simulink model "benchlink"  (R2024b)
settings: Solver=FixedStepDiscrete  StartTime=0.0  StopTime=0.005*16  RelTol=1e-3
model workspace (MAT data in the model file):
  socvcb : containers.Map (value not decoded)
values from neighbouring files (symbols this model uses):
  access = [32 0 4 36 32 0 4 36 32 0 4 36 ... (16 elements, 16x1)]    [all_variables.mat]
  qam_params =     [all_variables.mat]
undefined symbols (not defined in the file or in its folder): Add, j, QAM, rms, Shift
libraries: hdlsllib x53, simulink_need_slupdate x22, simulink x18, dspsigops x16, commdigbbndam3 x6, dsphdlmathfun2 x2, commchan3 x1, commrflib2 x1, dsphdlsigops2 x1, dspstat3 x1, dsphdlfiltering2 x1, simulink_extras x1
(part 2 of 5)

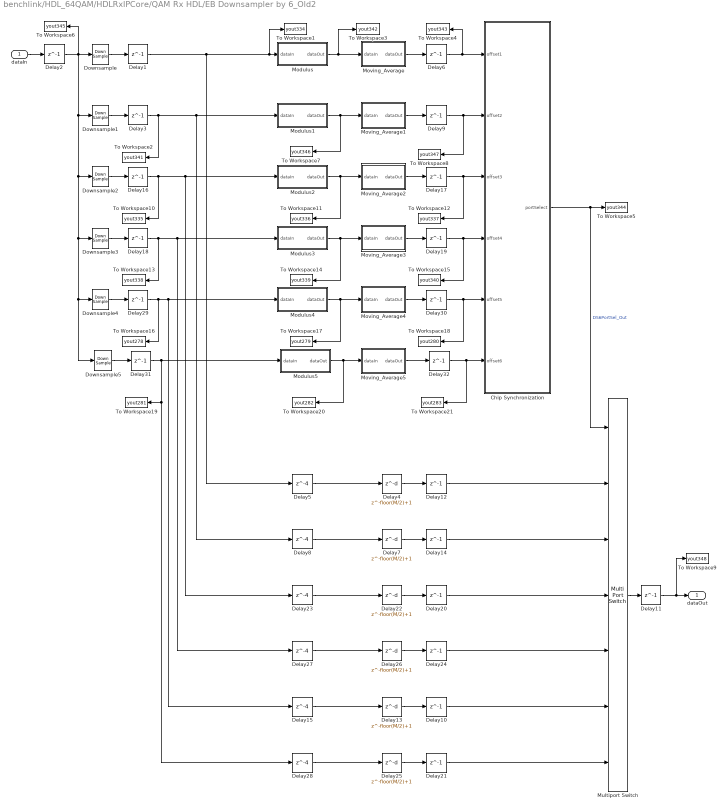
== system benchlink/HDL_64QAM/HDLRxIPCore/QAM Rx HDL/EB Downsampler by 6_Old2 ==
  dataIn : Inport  PortDimensions=1
  Chip Synchronization : MATLAB Function  TreatAsAtomicUnit=on
  Delay{1..3,6,9..12,14,16..21,24,29..32} (20 alike) : Delay  DelayLength=1  InitialCondition=0
  Delay{4,7,13,22,25..26} (6 alike) : Delay  DelayLength=floor(M/2)+1  InitialCondition=0
  Delay{5,8,15,23,27..28} (6 alike) : Delay  DelayLength=4  InitialCondition=0
  Downsample : DownSample  N=6  RateOptions=Allow multirate processing
  Downsample1 : DownSample  N=6  phase=1  RateOptions=Allow multirate processing
  Downsample2 : DownSample  N=6  phase=2  RateOptions=Allow multirate processing
  Downsample3 : DownSample  N=6  phase=3  RateOptions=Allow multirate processing
  Downsample4 : DownSample  N=6  phase=4  RateOptions=Allow multirate processing
  Downsample5 : DownSample  N=6  phase=5  RateOptions=Allow multirate processing
  Modulus : Subsystem
  Modulus1 : Subsystem
  Modulus2 : Subsystem
  Modulus3 : Subsystem
  Modulus4 : Subsystem
  Modulus5 : Subsystem
  Moving_Average : Subsystem
  Moving_Average1 : Subsystem
  Moving_Average2 : Subsystem
  Moving_Average3 : Subsystem
  Moving_Average4 : Subsystem
  Moving_Average5 : Subsystem
  Multiport Switch : MultiPortSwitch  Inputs=6  InputSameDT=off
  To Workspace1 : ToWorkspace  VariableName=yout334  SampleTime=-1
      settings: Save2DSignal=2-D array (concatenate along first dimension)
  To Workspace10 : ToWorkspace  VariableName=yout335  SampleTime=-1
      settings: Save2DSignal=2-D array (concatenate along first dimension)
  To Workspace11 : ToWorkspace  VariableName=yout336  SampleTime=-1
      settings: Save2DSignal=2-D array (concatenate along first dimension)
  To Workspace12 : ToWorkspace  VariableName=yout337  SampleTime=-1
      settings: Save2DSignal=2-D array (concatenate along first dimension)
  To Workspace13 : ToWorkspace  VariableName=yout338  SampleTime=-1
      settings: Save2DSignal=2-D array (concatenate along first dimension)
  To Workspace14 : ToWorkspace  VariableName=yout339  SampleTime=-1
      settings: Save2DSignal=2-D array (concatenate along first dimension)
  To Workspace15 : ToWorkspace  VariableName=yout340  SampleTime=-1
      settings: Save2DSignal=2-D array (concatenate along first dimension)
  To Workspace16 : ToWorkspace  VariableName=yout278  SampleTime=-1
      settings: Save2DSignal=2-D array (concatenate along first dimension)
  To Workspace17 : ToWorkspace  VariableName=yout279  SampleTime=-1
      settings: Save2DSignal=2-D array (concatenate along first dimension)
  To Workspace18 : ToWorkspace  VariableName=yout280  SampleTime=-1
      settings: Save2DSignal=2-D array (concatenate along first dimension)
  To Workspace19 : ToWorkspace  VariableName=yout281  SampleTime=-1
      settings: Save2DSignal=2-D array (concatenate along first dimension)
  To Workspace2 : ToWorkspace  VariableName=yout341  SampleTime=-1
      settings: Save2DSignal=2-D array (concatenate along first dimension)
  To Workspace20 : ToWorkspace  VariableName=yout282  SampleTime=-1
      settings: Save2DSignal=2-D array (concatenate along first dimension)
  To Workspace21 : ToWorkspace  VariableName=yout283  SampleTime=-1
      settings: Save2DSignal=2-D array (concatenate along first dimension)
  To Workspace3 : ToWorkspace  VariableName=yout342  SampleTime=-1
      settings: Save2DSignal=2-D array (concatenate along first dimension)
  To Workspace4 : ToWorkspace  VariableName=yout343  SampleTime=-1
      settings: Save2DSignal=2-D array (concatenate along first dimension)
  To Workspace5 : ToWorkspace  VariableName=yout344  SampleTime=-1
      settings: Save2DSignal=2-D array (concatenate along first dimension)
  To Workspace6 : ToWorkspace  VariableName=yout345  SampleTime=-1
      settings: Save2DSignal=2-D array (concatenate along first dimension)
  To Workspace7 : ToWorkspace  VariableName=yout346  SampleTime=-1
      settings: Save2DSignal=2-D array (concatenate along first dimension)
  To Workspace8 : ToWorkspace  VariableName=yout347  SampleTime=-1
      settings: Save2DSignal=2-D array (concatenate along first dimension)
  To Workspace9 : ToWorkspace  VariableName=yout348  SampleTime=-1
      settings: Save2DSignal=2-D array (concatenate along first dimension)
  dataOut : Outport  VectorParamsAs1DForOutWhenUnconnected=off
  wires:
  dataIn/1 -> Delay2/1
  Downsample/1 -> Delay1/1
  Modulus/1(dataOut) -> Moving_Average/1(dataIn), To Workspace3/1
  Modulus1/1(dataOut) -> Moving_Average1/1(dataIn), To Workspace7/1
  Moving_Average1/1(dataOut) -> Delay9/1
  Moving_Average/1(dataOut) -> Delay6/1
  Delay4/1 -> Delay12/1
  Delay5/1 -> Delay4/1
  Multiport Switch/1 -> Delay11/1
  Delay8/1 -> Delay7/1
  Downsample1/1 -> Delay3/1
  Delay7/1 -> Delay14/1
  Delay1/1 -> Delay5/1, To Workspace1/1, Modulus/1(dataIn)
  Delay3/1 -> To Workspace2/1, Delay8/1, Modulus1/1(dataIn)
  Delay6/1 -> To Workspace4/1, Chip Synchronization/1(offset1)
  Delay9/1 -> To Workspace8/1, Chip Synchronization/2(offset2)
  Chip Synchronization/1(portSelect) -> To Workspace5/1, Multiport Switch/1  "DS6PortSel_Out"
  Delay11/1 -> To Workspace9/1, dataOut/1
  Delay16/1 -> To Workspace10/1, Delay23/1, Modulus2/1(dataIn)
  Modulus2/1(dataOut) -> Moving_Average2/1(dataIn), To Workspace11/1
  Moving_Average2/1(dataOut) -> Delay17/1
  Delay17/1 -> To Workspace12/1, Chip Synchronization/3(offset3)
  Downsample2/1 -> Delay16/1
  Delay18/1 -> To Workspace13/1, Delay27/1, Modulus3/1(dataIn)
  Modulus3/1(dataOut) -> Moving_Average3/1(dataIn), To Workspace14/1
  Delay19/1 -> To Workspace15/1, Chip Synchronization/4(offset4)
  Downsample3/1 -> Delay18/1
  Moving_Average3/1(dataOut) -> Delay19/1
  Delay2/1 -> Downsample5/1, Downsample4/1, Downsample3/1, Downsample2/1, Downsample1/1, To Workspace6/1, Downsample/1
  Delay22/1 -> Delay20/1
  Delay23/1 -> Delay22/1
  Delay26/1 -> Delay24/1
  Delay27/1 -> Delay26/1
  Delay24/1 -> Multiport Switch/5
  Delay20/1 -> Multiport Switch/4
  Delay14/1 -> Multiport Switch/3
  Delay12/1 -> Multiport Switch/2
  Delay15/1 -> Delay13/1
  Delay13/1 -> Delay10/1
  Delay10/1 -> Multiport Switch/6
  Delay28/1 -> Delay25/1
  Delay25/1 -> Delay21/1
  Delay21/1 -> Multiport Switch/7
  Delay29/1 -> To Workspace16/1, Delay15/1, Modulus4/1(dataIn)
  Downsample4/1 -> Delay29/1
  Modulus4/1(dataOut) -> Moving_Average4/1(dataIn), To Workspace17/1
  Delay30/1 -> To Workspace18/1, Chip Synchronization/5(offset5)
  Moving_Average4/1(dataOut) -> Delay30/1
  Delay31/1 -> To Workspace19/1, Delay28/1, Modulus5/1(dataIn)
  Downsample5/1 -> Delay31/1
  Modulus5/1(dataOut) -> Moving_Average5/1(dataIn), To Workspace20/1
  Delay32/1 -> To Workspace21/1, Chip Synchronization/6(offset6)
  Moving_Average5/1(dataOut) -> Delay32/1

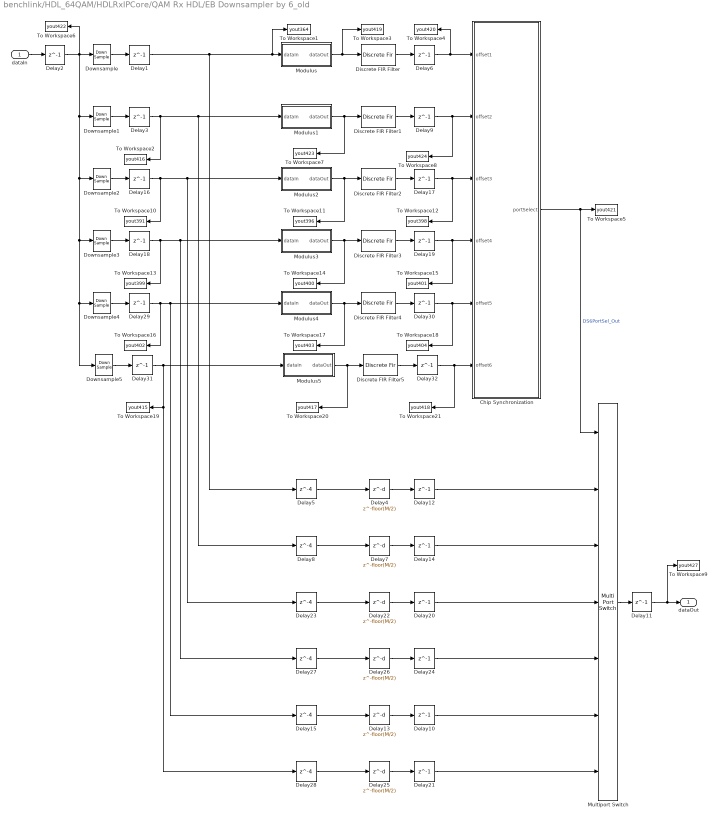
== system benchlink/HDL_64QAM/HDLRxIPCore/QAM Rx HDL/EB Downsampler by 6_old ==
  dataIn : Inport  PortDimensions=1
  Chip Synchronization : MATLAB Function  TreatAsAtomicUnit=on
  Delay{1..3,6,9..12,14,16..21,24,29..32} (20 alike) : Delay  DelayLength=1  InitialCondition=0
  Delay{4,7,13,22,25..26} (6 alike) : Delay  DelayLength=floor(M/2)  InitialCondition=0
  Delay{5,8,15,23,27..28} (6 alike) : Delay  DelayLength=4  InitialCondition=0
  Discrete FIR Filter{,1..5} (6 alike) : DiscreteFir  FilterStructure=Direct form transposed  Coefficients=ones(1,M)  CoefDataTypeStr=fixdt(1,2,0)  ProductDataTypeStr=fixdt(1,16,14)  AccumDataTypeStr=fixdt(1,16,16-floor(log2(M)+2))  OutDataTypeStr=fixdt(1,16,16-floor(log2(M)+2))  SaturateOnIntegerOverflow=on
  Downsample : DownSample  N=6  RateOptions=Allow multirate processing
  Downsample1 : DownSample  N=6  phase=1  RateOptions=Allow multirate processing
  Downsample2 : DownSample  N=6  phase=2  RateOptions=Allow multirate processing
  Downsample3 : DownSample  N=6  phase=3  RateOptions=Allow multirate processing
  Downsample4 : DownSample  N=6  phase=4  RateOptions=Allow multirate processing
  Downsample5 : DownSample  N=6  phase=5  RateOptions=Allow multirate processing
  Modulus : Subsystem
  Modulus1 : Subsystem
  Modulus2 : Subsystem
  Modulus3 : Subsystem
  Modulus4 : Subsystem
  Modulus5 : Subsystem
  Multiport Switch : MultiPortSwitch  Inputs=6  InputSameDT=off
  To Workspace1 : ToWorkspace  VariableName=yout364  SampleTime=-1
      settings: Save2DSignal=2-D array (concatenate along first dimension)
  To Workspace10 : ToWorkspace  VariableName=yout391  SampleTime=-1
      settings: Save2DSignal=2-D array (concatenate along first dimension)
  To Workspace11 : ToWorkspace  VariableName=yout396  SampleTime=-1
      settings: Save2DSignal=2-D array (concatenate along first dimension)
  To Workspace12 : ToWorkspace  VariableName=yout398  SampleTime=-1
      settings: Save2DSignal=2-D array (concatenate along first dimension)
  To Workspace13 : ToWorkspace  VariableName=yout399  SampleTime=-1
      settings: Save2DSignal=2-D array (concatenate along first dimension)
  To Workspace14 : ToWorkspace  VariableName=yout400  SampleTime=-1
      settings: Save2DSignal=2-D array (concatenate along first dimension)
  To Workspace15 : ToWorkspace  VariableName=yout401  SampleTime=-1
      settings: Save2DSignal=2-D array (concatenate along first dimension)
  To Workspace16 : ToWorkspace  VariableName=yout402  SampleTime=-1
      settings: Save2DSignal=2-D array (concatenate along first dimension)
  To Workspace17 : ToWorkspace  VariableName=yout403  SampleTime=-1
      settings: Save2DSignal=2-D array (concatenate along first dimension)
  To Workspace18 : ToWorkspace  VariableName=yout404  SampleTime=-1
      settings: Save2DSignal=2-D array (concatenate along first dimension)
  To Workspace19 : ToWorkspace  VariableName=yout415  SampleTime=-1
      settings: Save2DSignal=2-D array (concatenate along first dimension)
  To Workspace2 : ToWorkspace  VariableName=yout416  SampleTime=-1
      settings: Save2DSignal=2-D array (concatenate along first dimension)
  To Workspace20 : ToWorkspace  VariableName=yout417  SampleTime=-1
      settings: Save2DSignal=2-D array (concatenate along first dimension)
  To Workspace21 : ToWorkspace  VariableName=yout418  SampleTime=-1
      settings: Save2DSignal=2-D array (concatenate along first dimension)
  To Workspace3 : ToWorkspace  VariableName=yout419  SampleTime=-1
      settings: Save2DSignal=2-D array (concatenate along first dimension)
  To Workspace4 : ToWorkspace  VariableName=yout420  SampleTime=-1
      settings: Save2DSignal=2-D array (concatenate along first dimension)
  To Workspace5 : ToWorkspace  VariableName=yout421  SampleTime=-1
      settings: Save2DSignal=2-D array (concatenate along first dimension)
  To Workspace6 : ToWorkspace  VariableName=yout422  SampleTime=-1
      settings: Save2DSignal=2-D array (concatenate along first dimension)
  To Workspace7 : ToWorkspace  VariableName=yout423  SampleTime=-1
      settings: Save2DSignal=2-D array (concatenate along first dimension)
  To Workspace8 : ToWorkspace  VariableName=yout424  SampleTime=-1
      settings: Save2DSignal=2-D array (concatenate along first dimension)
  To Workspace9 : ToWorkspace  VariableName=yout427  SampleTime=-1
      settings: Save2DSignal=2-D array (concatenate along first dimension)
  dataOut : Outport  VectorParamsAs1DForOutWhenUnconnected=off
  wires:
  dataIn/1 -> Delay2/1
  Downsample/1 -> Delay1/1
  Modulus/1(dataOut) -> To Workspace3/1, Discrete FIR Filter/1
  Modulus1/1(dataOut) -> To Workspace7/1, Discrete FIR Filter1/1
  Discrete FIR Filter1/1 -> Delay9/1
  Discrete FIR Filter/1 -> Delay6/1
  Delay4/1 -> Delay12/1
  Delay5/1 -> Delay4/1
  Multiport Switch/1 -> Delay11/1
  Delay8/1 -> Delay7/1
  Downsample1/1 -> Delay3/1
  Delay7/1 -> Delay14/1
  Delay1/1 -> Delay5/1, To Workspace1/1, Modulus/1(dataIn)
  Delay3/1 -> To Workspace2/1, Delay8/1, Modulus1/1(dataIn)
  Delay6/1 -> To Workspace4/1, Chip Synchronization/1(offset1)
  Delay9/1 -> To Workspace8/1, Chip Synchronization/2(offset2)
  Chip Synchronization/1(portSelect) -> To Workspace5/1, Multiport Switch/1  "DS6PortSel_Out"
  Delay11/1 -> To Workspace9/1, dataOut/1
  Delay16/1 -> To Workspace10/1, Delay23/1, Modulus2/1(dataIn)
  Modulus2/1(dataOut) -> To Workspace11/1, Discrete FIR Filter2/1
  Discrete FIR Filter2/1 -> Delay17/1
  Delay17/1 -> To Workspace12/1, Chip Synchronization/3(offset3)
  Downsample2/1 -> Delay16/1
  Delay18/1 -> To Workspace13/1, Delay27/1, Modulus3/1(dataIn)
  Modulus3/1(dataOut) -> To Workspace14/1, Discrete FIR Filter3/1
  Delay19/1 -> To Workspace15/1, Chip Synchronization/4(offset4)
  Downsample3/1 -> Delay18/1
  Discrete FIR Filter3/1 -> Delay19/1
  Delay2/1 -> Downsample5/1, Downsample4/1, Downsample3/1, Downsample2/1, Downsample1/1, To Workspace6/1, Downsample/1
  Delay22/1 -> Delay20/1
  Delay23/1 -> Delay22/1
  Delay26/1 -> Delay24/1
  Delay27/1 -> Delay26/1
  Delay24/1 -> Multiport Switch/5
  Delay20/1 -> Multiport Switch/4
  Delay14/1 -> Multiport Switch/3
  Delay12/1 -> Multiport Switch/2
  Delay15/1 -> Delay13/1
  Delay13/1 -> Delay10/1
  Delay10/1 -> Multiport Switch/6
  Delay28/1 -> Delay25/1
  Delay25/1 -> Delay21/1
  Delay21/1 -> Multiport Switch/7
  Delay29/1 -> To Workspace16/1, Delay15/1, Modulus4/1(dataIn)
  Downsample4/1 -> Delay29/1
  Modulus4/1(dataOut) -> To Workspace17/1, Discrete FIR Filter4/1
  Delay30/1 -> To Workspace18/1, Chip Synchronization/5(offset5)
  Discrete FIR Filter4/1 -> Delay30/1
  Delay31/1 -> To Workspace19/1, Delay28/1, Modulus5/1(dataIn)
  Downsample5/1 -> Delay31/1
  Modulus5/1(dataOut) -> To Workspace20/1, Discrete FIR Filter5/1
  Delay32/1 -> To Workspace21/1, Chip Synchronization/6(offset6)
  Discrete FIR Filter5/1 -> Delay32/1

== system benchlink/HDL_64QAM/HDLRxIPCore/QAM Rx HDL/EQ Enable ==
  EQEnable : Inport
  Constant19 : Constant  OutDataTypeStr=boolean  SampleTime=1/(qam_params.chipRate)
  Constant20 : Constant  Value=0  OutDataTypeStr=boolean  SampleTime=1/(qam_params.chipRate)
  Switch9 : Switch  Criteria=u2 ~= 0  SaturateOnIntegerOverflow=off  InputSameDT=off
  Unit Delay : UnitDelay  InitialCondition=int16(150)  SampleTime=-1  HasFrameUpgradeWarning=on
  Out : Outport  VectorParamsAs1DForOutWhenUnconnected=off
  wires:
  EQEnable/1 -> Unit Delay/1
  Constant19/1 -> Switch9/1
  Unit Delay/1 -> Switch9/2
  Constant20/1 -> Switch9/3
  Switch9/1 -> Out/1

== system benchlink/HDL_64QAM/HDLRxIPCore/QAM Rx HDL/Enabled AGC1 ==
  x : Inport
  AGCEnable : Inport  Port=2  PortDimensions=1
  Constant : Constant  OutDataTypeStr=fixdt(1,24,15)  SampleTime=1/(qam_params.sampleRate)
  Delay : Delay  InitialCondition=0
  Delay1 : Delay  InitialCondition=0
  Delay2 : Delay  DelayLength=1  InitialCondition=0
  Delay3 : Delay  DelayLength=1  InitialCondition=0
  Delay4 : Delay  InitialCondition=0
  Energy Detector : Subsystem
  Loop gain : Constant  Value=AGC_Gain  OutDataTypeStr=fixdt(1,16,15)  SampleTime=1/qam_params.sampleRate
  Product : Product  OutDataTypeStr=fixdt(1,16,15)  SaturateOnIntegerOverflow=on
  Product1 : Product  OutDataTypeStr=fixdt(1,16,15)  SaturateOnIntegerOverflow=on
  Reference : Constant  Value=AGC_Ref  OutDataTypeStr=fixdt(1,16,15)  SampleTime=1/qam_params.sampleRate
  Sum : Sum  OutDataTypeStr=Inherit: Same as accumulator  AccumDataTypeStr=fixdt(1,24,15)  SaturateOnIntegerOverflow=on
  Sum1 : Sum  Inputs=|-+  OutDataTypeStr=Inherit: Same as first input
  Switch9 : Switch  Criteria=u2 ~= 0  SaturateOnIntegerOverflow=off  InputSameDT=off
  To Workspace1 : ToWorkspace  VariableName=yout471  SampleTime=-1
      settings: Save2DSignal=2-D array (concatenate along first dimension)
  To Workspace8 : ToWorkspace  VariableName=yout472  SampleTime=-1
      settings: Save2DSignal=2-D array (concatenate along first dimension)
  Unit Delay : UnitDelay  InitialCondition=.5  SampleTime=-1  HasFrameUpgradeWarning=on
  Unit Delay Enabled : simulink_need_slupdate/Unit Delay Enabled  vinit=1  tsamp=-1
  power : Subsystem
  gain : Outport  VectorParamsAs1DForOutWhenUnconnected=off
  y : Outport  Port=2  PortDimensions=1  VectorParamsAs1DForOutWhenUnconnected=off
  wires:
  Product/1 -> Delay/1
  Sum1/1 -> Delay2/1  "e"
  Delay2/1 -> Product1/1
  Product1/1 -> Delay4/1
  Unit Delay/1 -> gain/1, Switch9/1, Unit Delay Enabled/1  "g"
  Delay4/1 -> Sum/2
  x/1 -> Delay1/1
  Loop gain/1 -> Product1/2
  Sum/1 -> Unit Delay/1
  Reference/1 -> Sum1/2
  Delay1/1 -> To Workspace8/1, Product/1, Energy Detector/1(In)
  Delay/1 -> power/1(In1), y/1
  power/1(Out1) -> Sum1/1  "magnew"
  Energy Detector/1(Out) -> To Workspace1/1, Unit Delay Enabled/2
  Unit Delay Enabled/1 -> Sum/1
  Delay3/1 -> Switch9/2
  AGCEnable/1 -> Delay3/1
  Constant/1 -> Switch9/3
  Switch9/1 -> Product/2

== system benchlink/HDL_64QAM/HDLRxIPCore/QAM Rx HDL/Enabled AGC2 ==
  x : Inport
  AGCEnable : Inport  Port=2  PortDimensions=1
  Constant : Constant  OutDataTypeStr=fixdt(1,24,15)  SampleTime=1/(qam_params.sampleRate)
  Delay : Delay  InitialCondition=0
  Delay1 : Delay  InitialCondition=0
  Delay2 : Delay  DelayLength=1  InitialCondition=0
  Delay3 : Delay  DelayLength=1  InitialCondition=0
  Delay4 : Delay  InitialCondition=0
  Energy Detector : Subsystem
  Loop gain : Constant  Value=AGC_Gain  OutDataTypeStr=fixdt(1,16,15)  SampleTime=1/qam_params.sampleRate
  Product : Product  OutDataTypeStr=fixdt(1,16,15)  SaturateOnIntegerOverflow=on
  Product1 : Product  OutDataTypeStr=fixdt(1,16,15)  SaturateOnIntegerOverflow=on
  Reference : Constant  Value=AGC_Ref  OutDataTypeStr=fixdt(1,16,15)  SampleTime=1/qam_params.sampleRate
  Sum : Sum  OutDataTypeStr=Inherit: Same as accumulator  AccumDataTypeStr=fixdt(1,24,15)  SaturateOnIntegerOverflow=on
  Sum1 : Sum  Inputs=|-+  OutDataTypeStr=Inherit: Same as first input
  Switch9 : Switch  Criteria=u2 ~= 0  SaturateOnIntegerOverflow=off  InputSameDT=off
  Unit Delay : UnitDelay  InitialCondition=.5  SampleTime=-1  HasFrameUpgradeWarning=on
  Unit Delay Enabled : simulink_need_slupdate/Unit Delay Enabled  vinit=1  tsamp=-1
  power : Subsystem
  signal power1 : Subsystem
  gain : Outport  VectorParamsAs1DForOutWhenUnconnected=off
  y : Outport  Port=2  PortDimensions=1  VectorParamsAs1DForOutWhenUnconnected=off
  sig_power : Outport  Port=3  PortDimensions=1  VectorParamsAs1DForOutWhenUnconnected=off
  wires:
  Product/1 -> Delay/1
  Sum1/1 -> Delay2/1  "e"
  Delay2/1 -> Product1/1
  Product1/1 -> Delay4/1
  Delay4/1 -> Sum/2
  x/1 -> Delay1/1
  Loop gain/1 -> Product1/2
  Sum/1 -> Unit Delay/1
  Reference/1 -> Sum1/2
  Delay1/1 -> signal power1/1(x), Product/1, Energy Detector/1(In)
  Delay/1 -> power/1(In1), y/1
  power/1(Out1) -> Sum1/1  "magnew"
  Energy Detector/1(trigger) -> signal power1/2(trigger), Unit Delay Enabled/2
  Unit Delay Enabled/1 -> Sum/1
  AGCEnable/1 -> Delay3/1
  Delay3/1 -> Switch9/2
  Constant/1 -> Switch9/3
  Unit Delay/1 -> Unit Delay Enabled/1, Switch9/1, gain/1  "g"
  Switch9/1 -> Product/2
  signal power1/1(signal_power) -> sig_power/1

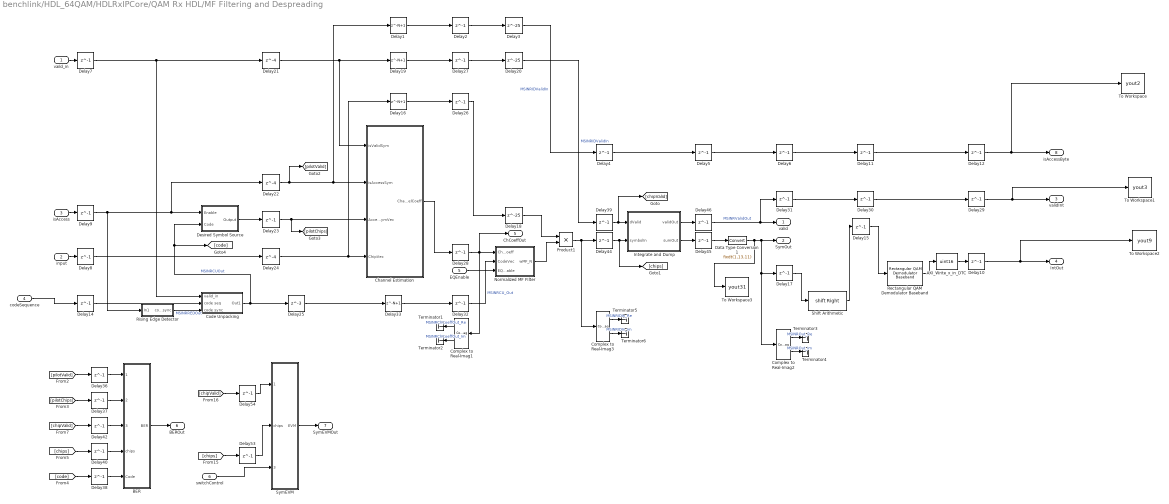
== system benchlink/HDL_64QAM/HDLRxIPCore/QAM Rx HDL/MF Filtering and Despreading ==
  vaild_in : Inport
  input : Inport  Port=2
  isAccess : Inport  Port=3
  codeSequence : Inport  Port=4
  EQEnable : Inport  Port=5
  switchControl : Inport  Port=6
  " Integrate and Dump" : MATLAB Function  TreatAsAtomicUnit=on
  AXI_Write_x_in_DTC : DataTypeConversion  OutDataTypeStr=uint16  ConvertRealWorld=Stored Integer (SI)  SaturateOnIntegerOverflow=off  RndMeth=Floor
  BER : Subsystem
  Channel Estimation : Subsystem
  Code Unpacking : Subsystem
  Complex to Real-Imag1 : ComplexToRealImag
  Complex to Real-Imag2 : ComplexToRealImag
  Complex to Real-Imag3 : ComplexToRealImag
  Data Type Conversion1 : DataTypeConversion  OutDataTypeStr=fixdt(1,13,11)  RndMeth=Floor
  Delay{1,16,19,33} (4 alike) : Delay  DelayLength=N+1  InitialCondition=0
  Delay{2,4..12,14..15,17,23,26..32,36..40,42,44..46,53..54} (32 alike) : Delay  DelayLength=1  InitialCondition=0
  Delay18 : Delay  DelayLength=25  InitialCondition=0
  Delay20 : Delay  DelayLength=25  InitialCondition=0
  Delay21 : Delay  DelayLength=4  InitialCondition=0
  Delay22 : Delay  DelayLength=4  InitialCondition=0
  Delay24 : Delay  DelayLength=4  InitialCondition=0
  Delay25 : Delay  DelayLength=3  InitialCondition=0
  Delay3 : Delay  DelayLength=25  InitialCondition=0
  Desired Symbol Source : Subsystem
  Normalized MF FIlter : Subsystem
  Product1 : Product  OutDataTypeStr=fixdt(1,16,14)  RndMeth=Zero  SaturateOnIntegerOverflow=on
  Rectangular QAM Demodulator Baseband : commdigbbndam3/Rectangular QAM Demodulator Baseband  M=64  OutType=Integer  DecType=Hard decision  VarSource=Dialog  Variance=1  Dec=Gray  Mapping=[0:15]  PowType=Min. distance between symbols  MinDist=2  AvgPow=0.66  PeakPow=1  Ph=0  outDtype1=boolean  outDtype2=Inherit via internal rule  derotateFactorWordLen=16  derotateFactorDataTypeStr=Inherit: Same word length as input  derotateFactorLastDataTypeStr=Inherit: Same word length as input  denormFactorWordLen=16  denormFactorDataTypeStr=Inherit: Same word length as input  denormFactorLastDataTypeStr=Inherit: Same word length as input  prodOutWordLen=32  prodOutOverflowMode=Wrap  prodOutRoundingMode=Floor  prodOutOvFlMode=off  prodOutOvFlModeLastStrValue=off  sumWordLen=32
  Rising Edge Detector : Subsystem
  Shift Arithmetic : ArithShift  BinPtShiftNumber=3  BitShiftDirection=Right
  SymEVM : Subsystem
  Terminator{1..6} (6 alike) : Terminator
  To Workspace : ToWorkspace  VariableName=yout2  SampleTime=-1
      settings: Save2DSignal=2-D array (concatenate along first dimension)
  To Workspace1 : ToWorkspace  VariableName=yout3  SampleTime=-1
      settings: Save2DSignal=2-D array (concatenate along first dimension)
  To Workspace2 : ToWorkspace  VariableName=yout9  SampleTime=-1
      settings: Save2DSignal=2-D array (concatenate along first dimension)
  To Workspace3 : ToWorkspace  VariableName=yout31  SampleTime=-1
      settings: Save2DSignal=2-D array (concatenate along first dimension)
  valid : Outport  InitialOutput=0  VectorParamsAs1DForOutWhenUnconnected=off
  SymOut : Outport  Port=2  InitialOutput=0  VectorParamsAs1DForOutWhenUnconnected=off
  validInt : Outport  Port=3  InitialOutput=0  VectorParamsAs1DForOutWhenUnconnected=off
  IntOut : Outport  Port=4  InitialOutput=0  VectorParamsAs1DForOutWhenUnconnected=off
  ChCoeffOut : Outport  Port=5  InitialOutput=0  VectorParamsAs1DForOutWhenUnconnected=off
  BEROut : Outport  Port=6  InitialOutput=0  VectorParamsAs1DForOutWhenUnconnected=off
  SymEVMOut : Outport  Port=7  InitialOutput=0  VectorParamsAs1DForOutWhenUnconnected=off
  isAccessByte : Outport  Port=8  InitialOutput=0  VectorParamsAs1DForOutWhenUnconnected=off
  wires:
  Delay14/1 -> Code Unpacking/2(code seq)
  vaild_in/1 -> Delay7/1
  input/1 -> Delay8/1
  codeSequence/1 -> Delay14/1
  isAccess/1 -> Delay9/1
  Desired Symbol Source/1(Output) -> Delay23/1
  Delay8/1 -> Delay24/1
  Delay9/1 -> Rising Edge Detector/1(In1), Desired Symbol Source/1(Enable), Delay22/1
  Channel Estimation/1(ChannelCoeff) -> Delay28/1
  Delay16/1 -> Delay26/1
  Code Unpacking/1(Out1) -> Delay25/1, [code], Desired Symbol Source/2(Code)  "MSINRCUOut"
  Delay19/1 -> Delay27/1
  Delay20/1 -> Delay39/1  "MSINRIDValidIn"
  Delay7/1 -> Code Unpacking/1(valid_in), Delay21/1
  Delay18/1 -> Product1/1
  Normalized MF FIlter/1(wMF_N) -> Product1/2
  Delay21/1 -> Delay19/1, Channel Estimation/1(isValidSym)
  Delay24/1 -> Delay16/1, Channel Estimation/4(ChipVec)
  Delay25/1 -> Delay33/1
  Delay26/1 -> Delay18/1
  Delay27/1 -> Delay20/1
  Delay28/1 -> ChCoeffOut/1, Complex to Real-Imag1/1, Normalized MF FIlter/1(ChannelCoeff)
  Shift Arithmetic/1 -> Delay15/1
  Delay15/1 -> Rectangular QAM Demodulator Baseband/1
  Rectangular QAM Demodulator Baseband/1 -> AXI_Write_x_in_DTC/1
  Delay17/1 -> Shift Arithmetic/1
  Delay10/1 -> To Workspace2/1, IntOut/1
  Delay29/1 -> To Workspace1/1, validInt/1
  Delay31/1 -> Delay30/1
  Delay30/1 -> Delay29/1
  Rising Edge Detector/1(code sync) -> Code Unpacking/3(code sync)  "MSINRREDOut"
  Delay45/1 -> Data Type Conversion1/1
  Product1/1 -> Complex to Real-Imag3/1, Delay44/1
  " Integrate and Dump"/1(validOut) -> Delay46/1
  " Integrate and Dump"/2(sumOut) -> Delay45/1
  Data Type Conversion1/1 -> To Workspace3/1, SymOut/1, Complex to Real-Imag2/1, Delay17/1
  Delay46/1 -> valid/1, Delay31/1  "MSINRValidOut"
  Delay32/1 -> Normalized MF FIlter/2(CodeVec)  "MSINRCU_Out"
  Complex to Real-Imag2/2 -> Terminator4/1  "MSINROut_Im"
  Complex to Real-Imag2/1 -> Terminator3/1  "MSINROut_Re"
  Complex to Real-Imag1/1 -> Terminator1/1  "MSINRChCoeffOut_Re"
  Complex to Real-Imag1/2 -> Terminator2/1  "MSINRChCoeffOut_Im"
  Complex to Real-Imag3/2 -> Terminator6/1  "MSINRIDIn_Im"
  Complex to Real-Imag3/1 -> Terminator5/1  "MSINRIDIn_Re"
  Delay33/1 -> Delay32/1
  EQEnable/1 -> Normalized MF FIlter/3(EQEnable)
  Delay54/1 -> SymEVM/1(chipValid)
  [chipValid] -> Delay54/1
  Delay53/1 -> SymEVM/2(chips)
  [pilotValid] -> Delay36/1
  [chips] -> Delay53/1
  Delay42/1 -> BER/3(chipValid)
  SymEVM/1(EVM) -> SymEVMOut/1
  [code] -> Delay38/1
  [pilotChips] -> Delay37/1
  Delay38/1 -> BER/5(Code)
  [chips] -> Delay40/1
  Delay37/1 -> BER/2(pilotChips)
  BER/1(BER) -> BEROut/1
  [chipValid] -> Delay42/1
  Delay40/1 -> BER/4(chips)
  Delay36/1 -> BER/1(pilotValid)
  Delay23/1 -> [pilotChips], Channel Estimation/3(AccessSymVec)
  Delay44/1 -> [chips], " Integrate and Dump"/2(symbolIn)
  Delay39/1 -> " Integrate and Dump"/1(dValid), [chipValid]
  Delay22/1 -> [pilotValid], Delay1/1, Channel Estimation/2(isAccessSym)
  AXI_Write_x_in_DTC/1 -> Delay10/1
  Delay1/1 -> Delay2/1
  Delay2/1 -> Delay3/1
  Delay3/1 -> Delay4/1  "MSINRIDValidIn"
  Delay4/1 -> Delay5/1
  Delay5/1 -> Delay6/1
  Delay6/1 -> Delay11/1
  Delay11/1 -> Delay12/1
  Delay12/1 -> To Workspace/1, isAccessByte/1
  switchControl/1 -> SymEVM/3(switchControl)

== system benchlink/HDL_64QAM/HDLRxIPCore/QAM Rx HDL/PD Threshold ==
  PDThreshold : Inport
  Bit Concat : hdlsllib/Logic and Bit Operations/Bit Concat  numInputs=7
  Bit Slice : hdlsllib/Logic and Bit Operations/Bit Slice  lidx=5  ridx=5
  Bit Slice1 : hdlsllib/Logic and Bit Operations/Bit Slice  lidx=4  ridx=4
  Bit Slice2 : hdlsllib/Logic and Bit Operations/Bit Slice  lidx=3  ridx=3
  Bit Slice3 : hdlsllib/Logic and Bit Operations/Bit Slice  lidx=2  ridx=2
  Bit Slice4 : hdlsllib/Logic and Bit Operations/Bit Slice  lidx=1  ridx=1
  Bit Slice5 : hdlsllib/Logic and Bit Operations/Bit Slice  lidx=0  ridx=0
  Bit Slice6 : hdlsllib/Logic and Bit Operations/Bit Slice  lidx=6  ridx=6
  Constant{6,8,10,12,14,16,18} (7 alike) : Constant  Value=0  OutDataTypeStr=boolean  SampleTime=1/(qam_params.chipRate)
  Constant{5,7,9,11,13,15,17} (7 alike) : Constant  OutDataTypeStr=boolean  SampleTime=1/(qam_params.chipRate)
  Scale : Gain  Gain=0.01  OutDataTypeStr=fixdt(0,16,15)  RndMeth=Zero
  Switch{1..7} (7 alike) : Switch  Criteria=u2 ~= 0  SaturateOnIntegerOverflow=off  InputSameDT=off
  Unit Delay : UnitDelay  InitialCondition=int16(150)  SampleTime=-1  HasFrameUpgradeWarning=on
  Out : Outport  VectorParamsAs1DForOutWhenUnconnected=off
  wires:
  Constant16/1 -> Switch6/3
  Bit Slice3/1 -> Switch5/2
  Constant17/1 -> Switch7/1
  Constant14/1 -> Switch5/3
  Bit Slice1/1 -> Switch3/2
  Constant13/1 -> Switch5/1
  Bit Slice4/1 -> Switch6/2
  Constant11/1 -> Switch4/1
  Bit Slice/1 -> Switch2/2
  Constant10/1 -> Switch3/3
  Bit Slice5/1 -> Switch7/2
  Bit Slice2/1 -> Switch4/2
  Constant18/1 -> Switch7/3
  Constant12/1 -> Switch4/3
  Constant6/1 -> Switch1/3
  Constant7/1 -> Switch2/1
  Constant15/1 -> Switch6/1
  Constant9/1 -> Switch3/1
  Bit Slice6/1 -> Switch1/2
  Constant5/1 -> Switch1/1
  Constant8/1 -> Switch2/3
  PDThreshold/1 -> Unit Delay/1
  Bit Concat/1 -> Scale/1
  Unit Delay/1 -> Bit Slice6/1, Bit Slice/1, Bit Slice1/1, Bit Slice2/1, Bit Slice3/1, Bit Slice4/1, Bit Slice5/1
  Scale/1 -> Out/1
  Switch1/1 -> Bit Concat/1
  Switch7/1 -> Bit Concat/7
  Switch6/1 -> Bit Concat/6
  Switch5/1 -> Bit Concat/5
  Switch4/1 -> Bit Concat/4
  Switch3/1 -> Bit Concat/3
  Switch2/1 -> Bit Concat/2

== system benchlink/HDL_64QAM/HDLRxIPCore/QAM Rx HDL/Payload Delimiter ==
  Input : Inport
  Threshold : Inport  Port=2
  fineCorrections : Inport  Port=3
  switchControl : Inport  Port=4
  packetSymLength : Inport  Port=5
  Constant : Constant  Commented=on  Value=threshold  OutDataTypeStr=Inherit: Inherit via back propagation  SampleTime=1/qam_params.chipRate
  Data Type Conversion1 : DataTypeConversion  RndMeth=Floor
  Delay{1..2,4..7,9..13} (11 alike) : Delay  DelayLength=1  InitialCondition=0
  For Normalized Modulus w Golay : Delay  DelayLength=7  InitialCondition=0
  MATLAB Function1 : MATLAB Function  TreatAsAtomicUnit=on
  MATLAB Function2 : MATLAB Function  Commented=on  TreatAsAtomicUnit=on
  Normalized Modulus : Subsystem
  Peak Detector : Subsystem
  Preamble Matched Filter : Subsystem
  Relational Operator : RelationalOperator  OutDataTypeStr=boolean
  Rising Edge Detector : Subsystem
  ffcControl : MATLAB Function  TreatAsAtomicUnit=on
  frameIndexing : Subsystem
  valid : Outport  InitialOutput=0  VectorParamsAs1DForOutWhenUnconnected=off
  output : Outport  Port=2  InitialOutput=0  VectorParamsAs1DForOutWhenUnconnected=off
  isAccess : Outport  Port=3  InitialOutput=0  VectorParamsAs1DForOutWhenUnconnected=off
  AccessStart : Outport  Port=4  InitialOutput=0  VectorParamsAs1DForOutWhenUnconnected=off
  wires:
  MATLAB Function1/1(isValid) -> Delay2/1
  MATLAB Function1/2(isAccess) -> Delay1/1
  Threshold/1 -> Data Type Conversion1/1
  Input/1 -> Delay12/1
  Delay2/1 -> valid/1
  Delay1/1 -> isAccess/1
  Delay11/1 -> output/1
  For Normalized Modulus w Golay/1 -> Delay5/1
  Delay9/1 -> Delay11/1
  Normalized Modulus/2(dataOutN) -> Relational Operator/1, Peak Detector/1(xCorr)  "PDNxCorrOut"
  Delay10/1 -> Delay4/1
  Delay4/1 -> AccessStart/1
  Preamble Matched Filter/1(dataOut) -> Normalized Modulus/1(dataIn)
  Relational Operator/1 -> Peak Detector/2(Threshold)
  Delay5/1 -> Delay13/1
  Data Type Conversion1/1 -> Relational Operator/2
  Peak Detector/1(Out1) -> Rising Edge Detector/1(In1), Delay6/1
  Delay6/1 -> MATLAB Function1/1(enable), Delay10/1
  Delay7/1 -> MATLAB Function1/2(count)
  Delay13/1 -> Delay9/1
  Delay12/1 -> Preamble Matched Filter/1(dataIn), For Normalized Modulus w Golay/1
  fineCorrections/1 -> ffcControl/1(correctionsPerPack)
  ffcControl/1(accessChipStart) -> MATLAB Function1/3(accessChipStart)
  Rising Edge Detector/1(Out1) -> frameIndexing/1(rst)
  frameIndexing/1(Out1) -> Delay7/1
  packetSymLength/1 -> MATLAB Function1/4(packetSymLen)
  switchControl/1 -> frameIndexing/2(switchControl), Normalized Modulus/2(switchControl)

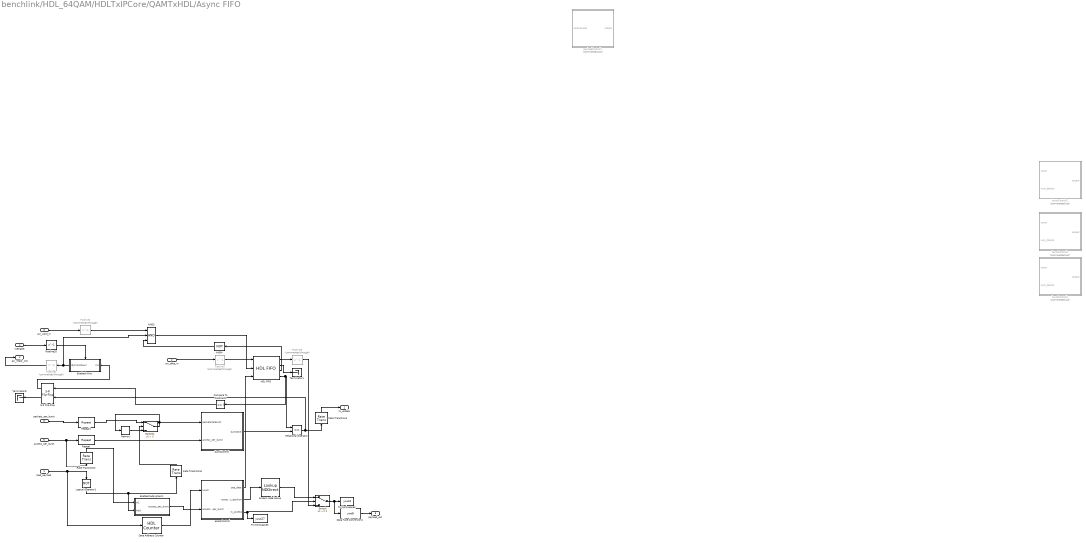
== system benchlink/HDL_64QAM/HDLTxIPCore/QAMTxHDL/Async FIFO ==
  load_payload : Inport
  axi_data_in : Inport  Port=2
  axi_valid_in : Inport  Port=3
  txEnable : Inport  Port=4
  access_per_burst : Inport  Port=5
  packets_per_burst : Inport  Port=6
  AND3 : Logic  Inputs=3  IconShape=distinctive  AllPortsSameDT=off  OutDataTypeStr=boolean
  AND4 : Logic  Operator=NOT  IconShape=distinctive  AllPortsSameDT=off  OutDataTypeStr=boolean
  Compare To Constant1 : simulink/Logic and Bit Operations/Compare To Constant  relop===  const=0  OutDataTypeStr=boolean
  Data Address Counter : hdlsllib/Sources/HDL Counter  CountType=Count limited  CountInit=0  CountStep=1  CountMax=255  CountFromType=Initial value  CountFrom=0  CountResetPort=off  CountLoadPort=off  CountEnbPort=on  CountDirPort=off  CountHitOutputPort=off  CountDataType=Unsigned  CountWordLen=16  CountFracLen=0  CountSampTime=1
  Data Type Conversion1 : DataTypeConversion  OutDataTypeStr=uint8  SaturateOnIntegerOverflow=off  RndMeth=Floor
  Enabled Subsystem1 : Subsystem  TreatAsAtomicUnit=on
  Enabled Wire : Subsystem  TreatAsAtomicUnit=on
  HDL FIFO : hdlsllib/HDL RAMs/HDL FIFO  fifo_size=2048  mode=Classic  ratio=48  push_msg=Warning  pop_msg=Warning  show_empty=on  show_full=on  show_num=on  LabelModeActiveChoice_Mode=Classic  rst_port=off
  Logical Operator1 : Logic  Operator=NOT  AllPortsSameDT=off  OutDataTypeStr=boolean
  Memory : Memory  InheritSampleTime=on
  Pipeline1 : Delay  Commented=through  DelayLength=1  InitialCondition=0  SampleTime=1/qam_params.sampleRate
  Pipeline2 : Delay  Commented=through  DelayLength=1  InitialCondition=0  SampleTime=1/qam_params.sampleRate
  Pipeline20 : Delay  DelayLength=1  InitialCondition=0
  Pipeline3 : Delay  Commented=through  DelayLength=1  InitialCondition=0  SampleTime=1/qam_params.sampleRate
  Pipeline9 : Delay  Commented=through  DelayLength=1  InitialCondition=0  SampleTime=1/qam_params.symbolRate
  Rate Transition1 : RateTransition  OutPortSampleTime=1/qam_params.symbolRate
  Rate Transition2 : RateTransition  OutPortSampleTime=1/qam_params.symbolRate
  Rate Transition3 : RateTransition  OutPortSampleTime=2.5000010000004e-08
  Relational Operator : RelationalOperator  Operator===  OutDataTypeStr=boolean  RndMeth=Simplest  InputSameDT=off
  Repeat : dspsigops/Repeat  FactorSource=Dialog parameter  N=qam_params.Upsampling  Nmax=16  InputProcessing=Columns as channels (frame based)  RateOptions=Allow multirate processing  ic=0  mode=Unused parameter value
  Repeat1 : dspsigops/Repeat  FactorSource=Dialog parameter  N=qam_params.Upsampling  Nmax=16  InputProcessing=Columns as channels (frame based)  RateOptions=Allow multirate processing  ic=0  mode=Unused parameter value
  S-R Flip-Flop : simulink_extras/Flip Flops/S-R Flip-Flop  initial_condition=0
  Switch : Switch  Criteria=u2 ~= 0  Threshold=15  SaturateOnIntegerOverflow=off  InputSameDT=off
  Switch1 : Switch  Criteria=u2 > Threshold  SaturateOnIntegerOverflow=off  InputSameDT=off
  Terminator1 : Terminator
  Terminator9 : Terminator
  To Workspace2 : ToWorkspace  VariableName=yout4  SampleTime=-1
      settings: Save2DSignal=2-D array (concatenate along first dimension)
  To Workspace3 : ToWorkspace  VariableName=yout27  SampleTime=-1
      settings: Save2DSignal=2-D array (concatenate along first dimension)
  access code lookup : LookupNDDirect  NumberOfTableDimensions=1  Table=access  DiagnosticForOutOfRangeInput=Error  TableDataTypeStr=uint32
  acessControl : MATLAB Function  TreatAsAtomicUnit=on
  burstControl : MATLAB Function  TreatAsAtomicUnit=on
  burstControl2 : MATLAB Function  Commented=on  TreatAsAtomicUnit=on
  burstControl3 : MATLAB Function  Commented=on  TreatAsAtomicUnit=on
  burstControl4 : MATLAB Function  Commented=on  TreatAsAtomicUnit=on
  payloadControl1 : MATLAB Function  Commented=on  TreatAsAtomicUnit=on  SystemSampleTime=1/qam_params.symbolRate
  tx_enable : Outport
  axi_ready_out : Outport  Port=2
  payload_out : Outport  Port=3
  wires:
  Enabled Wire/1(rdyFromDown) -> Pipeline1/1, AND3/2
  acessControl/3(is_access) -> Switch/2, To Workspace3/1
  Relational Operator/1 -> Rate Transition1/1, S-R Flip-Flop/2
  Compare To Constant1/1 -> S-R Flip-Flop/1
  Data Address Counter/1 -> acessControl/1(count)
  Pipeline3/1 -> HDL FIFO/1
  Pipeline2/1 -> AND3/1
  Pipeline1/1 -> axi_ready_out/1
  load_payload/1 -> Logical Operator1/1, Data Address Counter/1
  HDL FIFO/3 -> AND4/1
  Rate Transition1/1 -> tx_enable/1
  axi_valid_in/1 -> Pipeline2/1
  HDL FIFO/4 -> Compare To Constant1/1, Relational Operator/1
  S-R Flip-Flop/1 -> Enabled Wire/1(In1)
  axi_data_in/1 -> Pipeline3/1
  Switch/1 -> Data Type Conversion1/1, To Workspace2/1
  Rate Transition2/1 -> Enabled Subsystem1/1(In1)
  burstControl/1(burstSize) -> Relational Operator/2
  Repeat/1 -> burstControl/2(access_per_burst)
  acessControl/2(access_lut_position) -> access code lookup/1
  acessControl/1(pop_data) -> HDL FIFO/3
  Pipeline9/1 -> Switch/3
  HDL FIFO/2 -> Terminator1/1
  txEnable/1 -> Pipeline20/1
  Enabled Subsystem1/1(access_per_burst) -> acessControl/2(access_per_burst)
  access_per_burst/1 -> Rate Transition2/1, Repeat/1
  Logical Operator1/1 -> Rate Transition3/1, Enabled Subsystem1/2(hold)
  packets_per_burst/1 -> Repeat1/1
  Pipeline20/1 -> Enabled Wire/Enable
  access code lookup/1 -> Switch/1
  HDL FIFO/1 -> Pipeline9/1
  Data Type Conversion1/1 -> payload_out/1
  S-R Flip-Flop/2 -> Terminator9/1
  AND4/1 -> AND3/3
  AND3/1 -> HDL FIFO/2
  Repeat1/1 -> Switch1/1
  Switch1/1 -> burstControl/1(packetsPerBurst), Memory/1
  Rate Transition3/1 -> Switch1/2
  Memory/1 -> Switch1/3

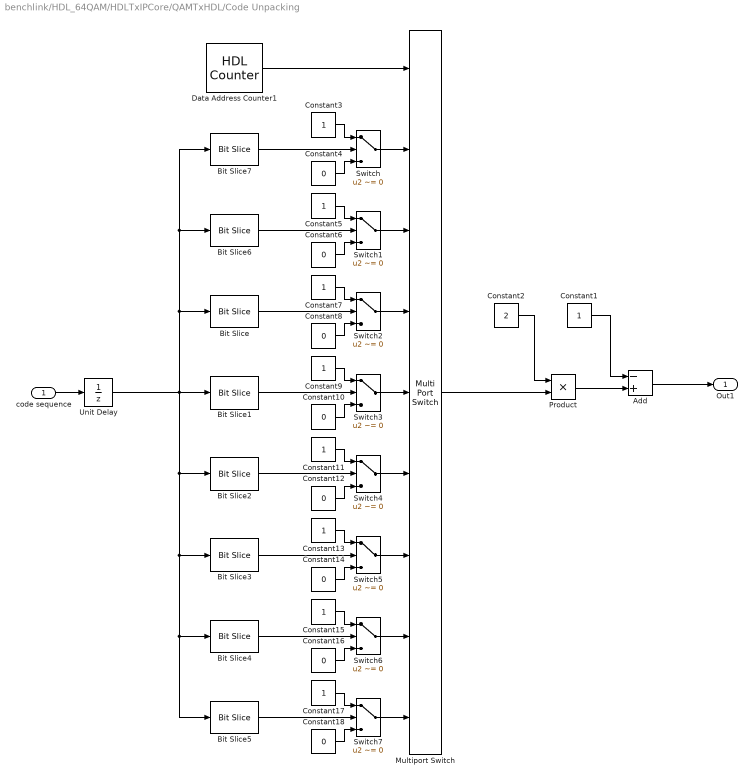
== system benchlink/HDL_64QAM/HDLTxIPCore/QAMTxHDL/Code Unpacking ==
  code sequence : Inport
  Add : Sum  Inputs=-+  OutDataTypeStr=fixdt(1,16,14)
  Bit Slice : hdlsllib/Logic and Bit Operations/Bit Slice  lidx=5  ridx=5
  Bit Slice1 : hdlsllib/Logic and Bit Operations/Bit Slice  lidx=4  ridx=4
  Bit Slice2 : hdlsllib/Logic and Bit Operations/Bit Slice  lidx=3  ridx=3
  Bit Slice3 : hdlsllib/Logic and Bit Operations/Bit Slice  lidx=2  ridx=2
  Bit Slice4 : hdlsllib/Logic and Bit Operations/Bit Slice  lidx=1  ridx=1
  Bit Slice5 : hdlsllib/Logic and Bit Operations/Bit Slice  lidx=0  ridx=0
  Bit Slice6 : hdlsllib/Logic and Bit Operations/Bit Slice  lidx=6  ridx=6
  Bit Slice7 : hdlsllib/Logic and Bit Operations/Bit Slice  lidx=7  ridx=7
  Constant1 : Constant  OutDataTypeStr=boolean  SampleTime=-1
  Constant{4,6,8,10,12,14,16,18} (8 alike) : Constant  Value=0  OutDataTypeStr=boolean  SampleTime=1/qam_params.chipRate
  Constant{3,5,7,9,11,13,15,17} (8 alike) : Constant  OutDataTypeStr=boolean  SampleTime=1/qam_params.chipRate
  Constant2 : Constant  Value=2  OutDataTypeStr=fixdt(1,16,0)  SampleTime=-1
  Data Address Counter1 : hdlsllib/Sources/HDL Counter  CountType=Count limited  CountInit=1  CountStep=1  CountMax=qam_params.spreadingFactor  CountFromType=Initial value  CountFrom=1  CountResetPort=off  CountLoadPort=off  CountEnbPort=off  CountDirPort=off  CountHitOutputPort=off  CountDataType=Unsigned  CountWordLen=16  CountFracLen=0  CountSampTime=1/qam_params.chipRate
  Multiport Switch : MultiPortSwitch  Inputs=8  SaturateOnIntegerOverflow=off  InputSameDT=off
  Product : Product
  Switch{,1..7} (8 alike) : Switch  Criteria=u2 ~= 0  SaturateOnIntegerOverflow=off  InputSameDT=off
  Unit Delay : UnitDelay  InitialCondition=int16(165)  SampleTime=-1  HasFrameUpgradeWarning=on
  Out1 : Outport  VectorParamsAs1DForOutWhenUnconnected=off
  wires:
  Product/1 -> Add/2
  Constant2/1 -> Product/1
  Constant1/1 -> Add/1
  Add/1 -> Out1/1
  Data Address Counter1/1 -> Multiport Switch/1
  Multiport Switch/1 -> Product/2
  code sequence/1 -> Unit Delay/1
  Unit Delay/1 -> Bit Slice5/1, Bit Slice4/1, Bit Slice3/1, Bit Slice2/1, Bit Slice7/1, Bit Slice6/1, Bit Slice/1, Bit Slice1/1
  Constant3/1 -> Switch/1
  Constant4/1 -> Switch/3
  Constant5/1 -> Switch1/1
  Constant6/1 -> Switch1/3
  Switch1/1 -> Multiport Switch/3
  Constant7/1 -> Switch2/1
  Constant8/1 -> Switch2/3
  Switch2/1 -> Multiport Switch/4
  Constant9/1 -> Switch3/1
  Constant10/1 -> Switch3/3
  Switch3/1 -> Multiport Switch/5
  Switch/1 -> Multiport Switch/2
  Constant11/1 -> Switch4/1
  Constant12/1 -> Switch4/3
  Switch4/1 -> Multiport Switch/6
  Constant13/1 -> Switch5/1
  Constant14/1 -> Switch5/3
  Switch5/1 -> Multiport Switch/7
  Constant15/1 -> Switch6/1
  Constant16/1 -> Switch6/3
  Switch6/1 -> Multiport Switch/8
  Constant17/1 -> Switch7/1
  Constant18/1 -> Switch7/3
  Switch7/1 -> Multiport Switch/9
  Bit Slice5/1 -> Switch7/2
  Bit Slice4/1 -> Switch6/2
  Bit Slice3/1 -> Switch5/2
  Bit Slice2/1 -> Switch4/2
  Bit Slice1/1 -> Switch3/2
  Bit Slice/1 -> Switch2/2
  Bit Slice6/1 -> Switch1/2
  Bit Slice7/1 -> Switch/2

== system benchlink/HDL_64QAM/HDLTxIPCore/QAMTxHDL/Enabled Subsystem ==
  In1 : Inport
  hold : Inport  Port=2
  Memory : Memory  InheritSampleTime=on
  Switch1 : Switch  Criteria=u2 > Threshold  SaturateOnIntegerOverflow=off  InputSameDT=off
  packetsPerBurst : Outport
  wires:
  Switch1/1 -> packetsPerBurst/1, Memory/1
  hold/1 -> Switch1/2
  In1/1 -> Switch1/1
  Memory/1 -> Switch1/3

== system benchlink/HDL_64QAM/HDLTxIPCore/QAMTxHDL/Packetization ==
  Reset Preamble : Inport
  Load Preamble : Inport  Port=2
  Data In : Inport  Port=3
  Code In : Inport  Port=4
  Pipeline1 : Delay  DelayLength=46  InitialCondition=0
  Pipeline2 : Delay  DelayLength=48  InitialCondition=0
  Pipeline3 : Delay  DelayLength=57  InitialCondition=0
  Pipeline4 : Delay  InitialCondition=0
  Pipeline5 : Delay  InitialCondition=0
  Pipeline6 : Delay  InitialCondition=0
  Preamble Address Counter : hdlsllib/Sources/HDL Counter  CountType=Count limited  CountInit=0  CountStep=1  CountMax=length(qam_params.preamble_symbols)-1  CountFromType=Initial value  CountFrom=0  CountResetPort=on  CountLoadPort=off  CountEnbPort=on  CountDirPort=off  CountHitOutputPort=off  CountDataType=Unsigned  CountWordLen=16  CountFracLen=0  CountSampTime=1
  Preamble Data Mux : Switch  Criteria=u2 ~= 0  SaturateOnIntegerOverflow=off  InputSameDT=off
  Product1 : Product  OutDataTypeStr=fixdt(1,16,15)  RndMeth=Zero
  Switch : Switch  Criteria=u2 > Threshold  Threshold=qam_params.golayLength  SaturateOnIntegerOverflow=off  InputSameDT=off
  Valid : Constant  OutDataTypeStr=boolean  SampleTime=1/qam_params.chipRate
  preamble lookup : LookupNDDirect  NumberOfTableDimensions=1  Table=qam_params.preamble_symbols  DiagnosticForOutOfRangeInput=Error  SampleTime=1/qam_params.chipRate  TableDataTypeStr=fixdt(1,16,15)
  Valid out : Outport  VectorParamsAs1DForOutWhenUnconnected=off
  Chip Out : Outport  Port=2  VectorParamsAs1DForOutWhenUnconnected=off
  wires:
  Load Preamble/1 -> Pipeline2/1, Preamble Address Counter/2
  Reset Preamble/1 -> Preamble Address Counter/1
  Preamble Address Counter/1 -> Pipeline5/1, preamble lookup/1
  Preamble Data Mux/1 -> Chip Out/1
  Data In/1 -> Preamble Data Mux/3
  Pipeline1/1 -> Preamble Data Mux/1
  Pipeline2/1 -> Preamble Data Mux/2
  Valid/1 -> Pipeline3/1
  Pipeline3/1 -> Valid out/1
  Code In/1 -> Product1/1
  Product1/1 -> Pipeline4/1
  Pipeline4/1 -> Switch/1
  Pipeline5/1 -> Switch/2
  Pipeline6/1 -> Switch/3
  preamble lookup/1 -> Product1/2, Pipeline6/1
  Switch/1 -> Pipeline1/1

== system benchlink/HDL_64QAM/HDLTxIPCore/QAMTxHDL/Pulse Shaping ==
  dataIn : Inport
  RRC Interpolation Filter : dspmlti4/FIR Interpolation  FilterSource=Dialog parameters  PrivateCoeffs=0  h=qam_params.TransmitterFilterCoefficients  L=qam_params.Upsampling  FilterObject=Htxrc  framing=Allow multirate processing  outputBufInitCond=0  roundingMode=Nearest  overflowMode=on  firstCoeffMode=Binary point scaling  firstCoeffWordLength=16  firstCoeffFracLength=15  firstCoeffDataTypeStr=fixdt(1,16,15)  firstCoeffMin=[]  firstCoeffMax=[]  firstCoeffLastDataTypeStr=fixdt(1,16,15)  outputMode=Binary point scaling  outputWordLength=16  outputFracLength=15  outputDataTypeStr=fixdt(1,16,15)  outputMin=[]  outputMax=[]  outputLastDataTypeStr=fixdt(1,16,15)
  dataOut : Outport  VectorParamsAs1DForOutWhenUnconnected=off
  wires:
  RRC Interpolation Filter/1 -> dataOut/1
  dataIn/1 -> RRC Interpolation Filter/1

== system benchlink/HDL_64QAM/HDLTxIPCore/QAMTxHDL/Subsystem2 ==
  txEnable : Inport
  Edge Detector : Subsystem
  HDL Counter : hdlsllib/Sources/HDL Counter  CountType=Count limited  CountInit=0  CountStep=1  CountMax=1  CountFromType=Initial value  CountFrom=0  CountResetPort=off  CountLoadPort=off  CountEnbPort=on  CountDirPort=off  CountHitOutputPort=off  CountDataType=Unsigned  CountWordLen=1  CountFracLen=0  CountSampTime=-1
  Rate Transition : RateTransition  InitialCondition=true  OutPortSampleTime=1/qam_params.symbolRate
  transmitNow : Outport  VectorParamsAs1DForOutWhenUnconnected=off
  wires:
  txEnable/1 -> HDL Counter/1
  HDL Counter/1 -> Rate Transition/1
  Edge Detector/1(Out1) -> transmitNow/1
  Rate Transition/1 -> Edge Detector/1(In1)

== system benchlink/HDL_64QAM/HDLTxIPCore/QAMTxHDL/Symbol Mapping ==
  Valid In : Inport
  Integer In : Inport  Port=2
  Rectangular QAM Modulator Baseband : commdigbbndam3/Rectangular QAM Modulator Baseband  M=64  InType=Integer  Enc=Gray  Mapping=[0:15]  PowType=Min. distance between symbols  MinDist=0.25  AvgPow=.66  PeakPow=1.1  Ph=0  outDtype=Fixed-point  outWordLen=16  outUDDataType=sfix(16)  outFracLenMode=Best precision  outFracLen=15  outDataTypeStr=fixdt(1,16)  outLastDataTypeStr=fixdt(1,16)
  Valid out : Outport  VectorParamsAs1DForOutWhenUnconnected=off
  Symbol Out : Outport  Port=2  VectorParamsAs1DForOutWhenUnconnected=off
  wires:
  Rectangular QAM Modulator Baseband/1 -> Symbol Out/1
  Integer In/1 -> Rectangular QAM Modulator Baseband/1
  Valid In/1 -> Valid out/1

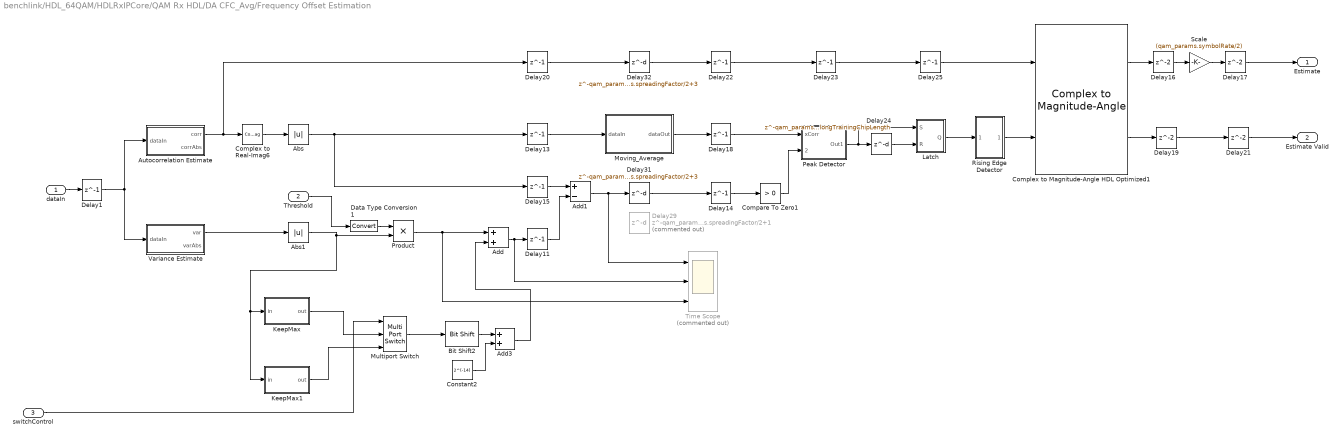
== system benchlink/HDL_64QAM/HDLRxIPCore/QAM Rx HDL/DA CFC_Avg/Frequency Offset Estimation ==
  dataIn : Inport
  Threshold : Inport  Port=2
  switchControl : Inport  Port=3
  Abs : Abs
  Abs1 : Abs
  Add : Sum  OutDataTypeStr=fixdt(1,32,20)
  Add1 : Sum  Inputs=+-  OutDataTypeStr=fixdt(1,64,46)  AccumDataTypeStr=fixdt(1,64,46)
  Add3 : Sum  OutDataTypeStr=fixdt(0,8,8)  SaturateOnIntegerOverflow=on
  Autocorrelation Estimate : Subsystem
  Bit Shift2 : hdlsllib/Logic and Bit Operations/Bit Shift  mode=Shift Right Arithmetic  N=4
  Compare To Zero1 : simulink/Logic and Bit Operations/Compare To Zero  relop=>  OutDataTypeStr=boolean
  Complex to Real-Imag6 : ComplexToRealImag  Output=Real
  Complex to Magnitude-Angle HDL Optimized1 : dsphdlmathfun2/Complex to Magnitude-Angle  NumIterationsSource=Auto  NumIterations=10  OutputFormat=Angle  AngleFormat=Normalized  ScaleOutput=on  ScalingMethod=Shift-Add  SimulateUsing=Code generation
  Constant2 : Constant  Value=2^(-14)  OutDataTypeStr=fixdt(0,16,14)  SampleTime=-1
  Data Type Conversion1 : DataTypeConversion  RndMeth=Floor
  Delay{1,11,13..15,18,20,22..23,25} (10 alike) : Delay  DelayLength=1  InitialCondition=0  UseCircularBuffer=on
  Delay{16..17,19,21} (4 alike) : Delay  InitialCondition=0  UseCircularBuffer=on
  Delay24 : Delay  DelayLength=qam_params.longTrainingChipLength  InitialCondition=0  UseCircularBuffer=on
  Delay29 : Delay  Commented=on  DelayLength=qam_params.spreadingFactor/2+1  InitialCondition=0  UseCircularBuffer=on
  Delay31 : Delay  DelayLength=qam_params.spreadingFactor/2+3  InitialCondition=0  UseCircularBuffer=on
  Delay32 : Delay  DelayLength=qam_params.spreadingFactor/2+3  InitialCondition=0  UseCircularBuffer=on
  KeepMax : MATLAB Function  TreatAsAtomicUnit=on
  KeepMax1 : MATLAB Function  TreatAsAtomicUnit=on
  Latch : Subsystem
  Moving_Average : Subsystem
  Multiport Switch : MultiPortSwitch  Inputs=2  SaturateOnIntegerOverflow=off  InputSameDT=off
  Peak Detector : Subsystem
  Product : Product
  Rising Edge Detector : Subsystem
  Scale : Gain  Gain=(qam_params.symbolRate/2)  OutDataTypeStr=int16  RndMeth=Zero
  Time Scope : Scope  Commented=on  NumInputPorts=3
  Variance Estimate : Subsystem
  Estimate : Outport  VectorParamsAs1DForOutWhenUnconnected=off
  Estimate Valid : Outport  Port=2  VectorParamsAs1DForOutWhenUnconnected=off
  wires:
  Rising Edge Detector/1(Out1) -> Complex to Magnitude-Angle HDL Optimized1/2
  Variance Estimate/1(var) -> Abs1/1
  Add/1 -> Time Scope/2, Delay11/1
  Delay31/1 -> Delay14/1
  Moving_Average/1(dataOut) -> Delay18/1
  Delay32/1 -> Delay22/1
  Delay13/1 -> Moving_Average/1(dataIn)
  Abs/1 -> Delay15/1, Delay13/1
  Latch/1(Q) -> Rising Edge Detector/1(In1)
  Complex to Real-Imag6/1 -> Abs/1
  Abs1/1 -> KeepMax1/1(in), KeepMax/1(in), Product/2
  Delay11/1 -> Add1/2
  Delay22/1 -> Delay23/1
  Complex to Magnitude-Angle HDL Optimized1/1 -> Delay16/1
  Bit Shift2/1 -> Add3/1
  Add1/1 -> Time Scope/1, Delay31/1
  Delay23/1 -> Delay25/1
  Delay14/1 -> Compare To Zero1/1
  Delay24/1 -> Latch/2(R)
  Delay20/1 -> Delay32/1
  Add3/1 -> Add/2
  Peak Detector/1(Out1) -> Delay24/1, Latch/1(S)
  Delay18/1 -> Peak Detector/1(xCorr)
  Compare To Zero1/1 -> Peak Detector/2(Threshold)
  KeepMax/1(out) -> Multiport Switch/2
  Autocorrelation Estimate/1(corr) -> Delay20/1, Complex to Real-Imag6/1
  Constant2/1 -> Add3/2
  Product/1 -> Time Scope/3, Add/1
  Delay15/1 -> Add1/1
  Delay16/1 -> Scale/1
  Scale/1 -> Delay17/1
  Complex to Magnitude-Angle HDL Optimized1/2 -> Delay19/1
  Delay19/1 -> Delay21/1
  Delay25/1 -> Complex to Magnitude-Angle HDL Optimized1/1
  Delay21/1 -> Estimate Valid/1
  Delay17/1 -> Estimate/1
  dataIn/1 -> Delay1/1
  Delay1/1 -> Autocorrelation Estimate/1(dataIn), Variance Estimate/1(dataIn)
  Threshold/1 -> Data Type Conversion1/1
  Data Type Conversion1/1 -> Product/1
  switchControl/1 -> Multiport Switch/1
  KeepMax1/1(out) -> Multiport Switch/3
  Multiport Switch/1 -> Bit Shift2/1
